simulink model "Greenhouse_Active_Passive_Solar_final"  (R2020b)
settings: Solver=VariableStepAuto  StartTime=0.0  StopTime=8759  RelTol=1e-3
libraries: simulink x1
settings Model: Creator=jkarenzi  LastModifiedBy=michelechamberlin

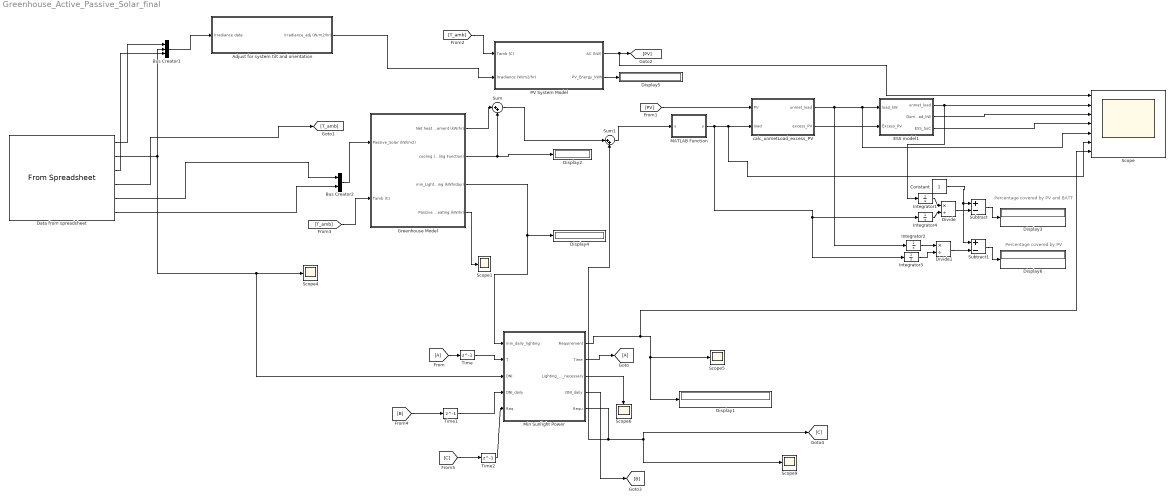
== system Greenhouse_Active_Passive_Solar_final ==
  note: Percentage covered by PV
  note: Percentage covered by PV and BATT
  Adjust for system tilt and orientation : Subsystem  TreatAsAtomicUnit=on  mask{P1=65, P2=65, P3=180}
      mask prompts: P1 "Latitude (degrees)"; P2 "System tilt (degrees)"; P3 "System Orientation (degrees)"
      mask init:
      | L = P1;
      | B = P2;
      | Z = P3;
  Bus Creator1 : BusCreator  Inputs=3
  Bus Creator2 : BusCreator  Inputs=2
  Constant : Constant
  Data from spreadsheet : FromSpreadsheet  FileName=C:\Users\michelechamberlin\Desktop\MicroFEWs\MATLAB Simulink\Tanana\GreenhouseData.xlsx  SheetName=GreenhouseData  Range=A1:G8761  SampleTime=1
  Display{1..6} (6 alike) : Display
  Divide : Product  Inputs=*/
  Divide1 : Product  Inputs=*/
  ESS model1 : Subsystem  TreatAsAtomicUnit=on  mask{P1=100, P2=100, P3=30, P4=90, P5=80}
      mask prompts: P1 "ESS Capacity"; P2 "Initial_SoC (%)"; P3 "Min_SoC (%)"; P4 "Max_SoC (%)"; P5 "Battery Efficieny (%)"
      mask init:
      | Bat_capacity = P1;
      | Init_SoC = P2;
      | min_SoC = P3;
      | max_SoC = P4;
      | bat_eff = P5;
  Greenhouse Model : Subsystem  mask{P1=60, P2=16, P3=750}
      mask prompts: P1 "Minimum inside temperature (F)"; P2 "Daily Artificial Lighting Hours"; P3 "Min. lighting requirements (fc)"
      mask init:
      | %Initialization
      | Tin = P1;
      | AL_hrs = P2;
      | min_lighting = P3;
  Integrator{1..4} (4 alike) : Integrator
  MATLAB Function : MATLAB Function  TreatAsAtomicUnit=on
  Min Sunlight Power : MATLAB Function  TreatAsAtomicUnit=on
  PV System Model : Subsystem  mask{DC=10, TC=-0.0037, MM=15, Inv=96}
      mask prompts: DC "DC system size (kW)"; TC "Temp coeff (%)"; MM "System losses (%)"; Inv "Inverter efficiency (%)"
      mask init:
      | %initiliaze the parameters
      | %PV System size
      | DC_kW = DC; %DC system size
      | T_coeff = TC; %temp coefficient
      | 
      | %define losses
      | L_modules = MM; %losses due to module mismatch
      | %L_dirt = LD; %Losses due to dirt
      | 
      | inv_eff = Inv; %inverter efficiency
  Scope : Scope  NumInputPorts=7
  Scope{1,4..6,9} (5 alike) : Scope
  Subtract : Sum  Inputs=+-
  Subtract1 : Sum  Inputs=+-
  Sum : Sum  Inputs=|++
  Sum1 : Sum  Inputs=|++
  Time : Delay  DelayLength=1  InitialCondition=0  SampleTime=1
  Time1 : Delay  DelayLength=1  InitialCondition=0  SampleTime=1
  Time2 : Delay  DelayLength=1  InitialCondition=0  SampleTime=1
  calc_unmetLoad_excess_PV : MATLAB Function  TreatAsAtomicUnit=on
  wires:
  Greenhouse Model/2(cooling (m3/s/m2) NEW: kW (Check cooling Function)) -> Sum/2, Display2/1
  Greenhouse Model/3(min_Lighting (kWh/day)) -> Min Sunlight Power/1(min_daily_lighting), Display4/1
  Bus Creator1/1 -> Adjust for system tilt and orientation/1(Irradiance data)
  Adjust for system tilt and orientation/1(Irradiance_adj (W/m2/hr)) -> PV System Model/2(Irradiance (W/m2/hr))
  PV System Model/2(PV_Energy_kWh) -> Display5/1
  PV System Model/1(AC (kW)) -> Scope/1, [PV]
  Data from spreadsheet/6 -> Bus Creator2/2
  Data from spreadsheet/5 -> Bus Creator2/1
  Data from spreadsheet/1 -> Bus Creator1/1
  Data from spreadsheet/2 -> Min Sunlight Power/3(DNI), Scope4/1, Bus Creator1/2
  Data from spreadsheet/3 -> Bus Creator1/3
  Data from spreadsheet/4 -> [T_amb]
  [T_amb] -> PV System Model/1(Tamb (C))
  Bus Creator2/1 -> Greenhouse Model/1(Passive_Solar (kW/m2))
  [T_amb] -> Greenhouse Model/2(Tamb (C))
  Greenhouse Model/4(Passive heating (kW/hr)) -> Scope1/1
  ESS model1/1(unmet_load) -> Integrator1/1, Scope/2
  [PV] -> calc_unmetLoad_excess_PV/1(PV)
  calc_unmetLoad_excess_PV/2(excess_PV) -> ESS model1/2(Excess_PV)
  Greenhouse Model/1(Net heat requirement (kW/hr)) -> Sum/1
  ESS model1/2(Dump_load_kW) -> Scope/3
  ESS model1/3(ESS_SoC) -> Scope/4
  Min Sunlight Power/1(Requirement) -> Display1/1, Scope5/1, Scope/7
  Min Sunlight Power/3(Lighting_Wh_necessary) -> Scope6/1
  [A] -> Time/1
  Time/1 -> Min Sunlight Power/2(T)
  Min Sunlight Power/2(Time) -> [A]
  Sum1/1 -> MATLAB Function/1(u)
  Sum/1 -> Sum1/1
  MATLAB Function/1(y) -> Integrator3/1, Integrator4/1, Scope/6, calc_unmetLoad_excess_PV/2(load)
  Integrator1/1 -> Divide/1
  Integrator4/1 -> Divide/2
  Divide/1 -> Subtract/2
  Integrator2/1 -> Divide1/1
  Divide1/1 -> Subtract1/2
  Integrator3/1 -> Divide1/2
  calc_unmetLoad_excess_PV/1(unmet_load) -> Integrator2/1, Scope/5, ESS model1/1(load_kW)
  Constant/1 -> Subtract/1, Subtract1/1
  Subtract/1 -> Display3/1
  Subtract1/1 -> Display6/1
  Min Sunlight Power/4(DNI_daily) -> [B]
  [B] -> Time1/1
  Time1/1 -> Min Sunlight Power/4("DNI_daily ")
  Time2/1 -> Min Sunlight Power/5(Req)
  [C] -> Time2/1
  Min Sunlight Power/5(Requ) -> Scope9/1, [C], Sum1/2

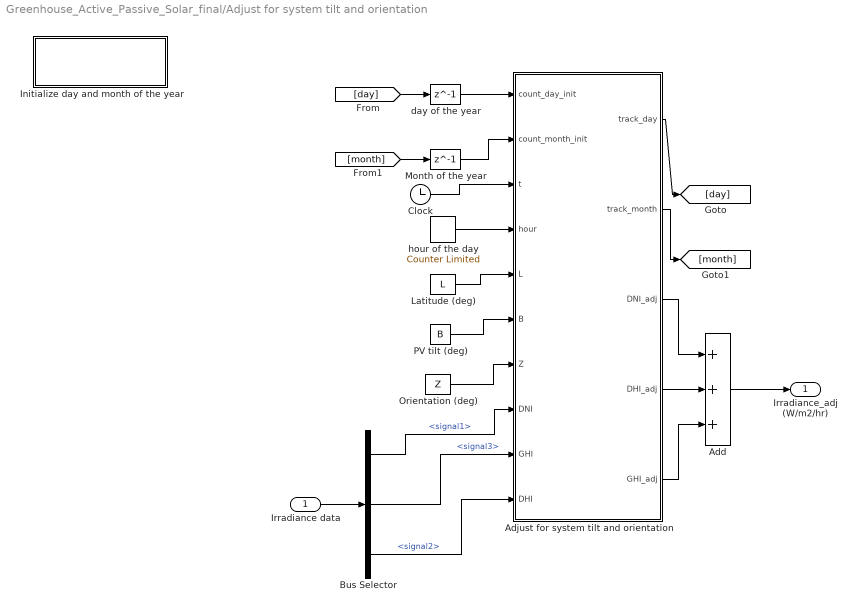
== system Greenhouse_Active_Passive_Solar_final/Adjust for system tilt and orientation ==
  Irradiance data : Inport
  Add : Sum  Inputs=+++
  Adjust for system tilt and orientation : MATLAB Function  TreatAsAtomicUnit=on
  Bus Selector : BusSelector  OutputSignals=signal1,signal3,signal2
  Clock : Clock
  Initialize day and month of the year : Subsystem  TreatAsAtomicUnit=on
  Latitude (deg) : Constant  Value=L
  Month of the year : Delay  DelayLength=1  InitialCondition=0  SampleTime=1
  Orientation (deg) : Constant  Value=Z
  PV tilt (deg) : Constant  Value=B
  day of the year : Delay  DelayLength=1  InitialCondition=0  SampleTime=1
  hour of the day : simulink/Sources/Counter Limited  uplimit=24  tsamp=1
  Irradiance_adj (W/m2/hr) : Outport
  wires:
  [month] -> Month of the year/1
  Adjust for system tilt and orientation/1(track_day) -> [day]
  Adjust for system tilt and orientation/5(GHI_adj) -> Add/3
  day of the year/1 -> Adjust for system tilt and orientation/1(count_day_init)
  PV tilt (deg)/1 -> Adjust for system tilt and orientation/6(B)
  Month of the year/1 -> Adjust for system tilt and orientation/2(count_month_init)
  Adjust for system tilt and orientation/2(track_month) -> [month]
  hour of the day/1 -> Adjust for system tilt and orientation/4(hour)
  Clock/1 -> Adjust for system tilt and orientation/3(t)
  [day] -> day of the year/1
  Orientation (deg)/1 -> Adjust for system tilt and orientation/7(Z)
  Adjust for system tilt and orientation/3(DNI_adj) -> Add/1
  Adjust for system tilt and orientation/4(DHI_adj) -> Add/2
  Latitude (deg)/1 -> Adjust for system tilt and orientation/5(L)
  Add/1 -> Irradiance_adj (W/m2/hr)/1
  Irradiance data/1 -> Bus Selector/1
  Bus Selector/1 -> Adjust for system tilt and orientation/8(DNI)  "<signal1>"
  Bus Selector/2 -> Adjust for system tilt and orientation/9(GHI)  "<signal3>"
  Bus Selector/3 -> Adjust for system tilt and orientation/10(DHI)  "<signal2>"

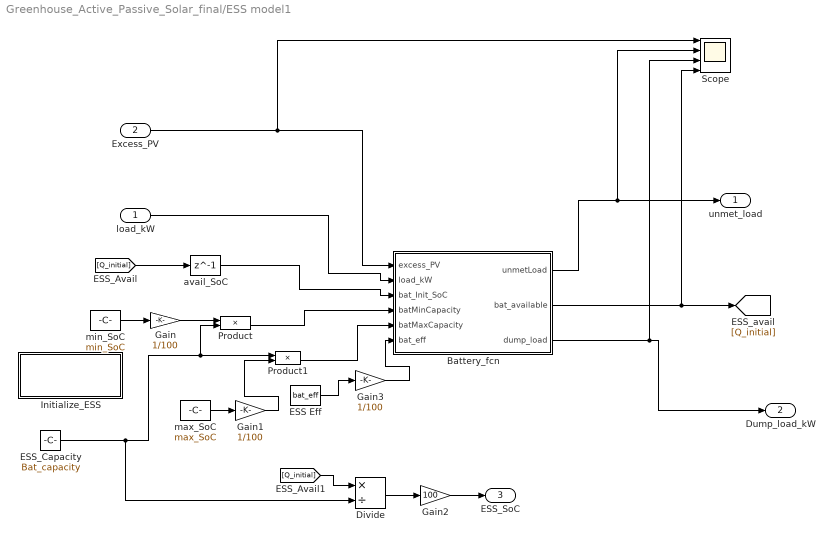
== system Greenhouse_Active_Passive_Solar_final/ESS model1 ==
  load_kW : Inport
  Excess_PV : Inport  Port=2
  Battery_fcn : MATLAB Function  TreatAsAtomicUnit=on
  Divide : Product  Inputs=*/
  ESS Eff : Constant  Value=bat_eff
  "ESS_Capacity " : Constant  Value=Bat_capacity
  Gain : Gain  Gain=1/100
  Gain1 : Gain  Gain=1/100
  Gain2 : Gain  Gain=100
  Gain3 : Gain  Gain=1/100
  Initialize_ESS : Subsystem  TreatAsAtomicUnit=on
  Product : Product
  Product1 : Product
  Scope : Scope  NumInputPorts=4
  avail_SoC : Delay  DelayLength=1  InitialCondition=0  SampleTime=1
  max_SoC : Constant  Value=max_SoC
  min_SoC : Constant  Value=min_SoC
  unmet_load : Outport
  Dump_load_kW : Outport  Port=2
  ESS_SoC : Outport  Port=3
  wires:
  Excess_PV/1 -> Scope/1, Battery_fcn/1(excess_PV)
  avail_SoC/1 -> Battery_fcn/3(bat_Init_SoC)
  Battery_fcn/1(unmetLoad) -> Scope/2, unmet_load/1
  [Q_initial] -> avail_SoC/1
  max_SoC/1 -> Gain1/1
  min_SoC/1 -> Gain/1
  Gain/1 -> Product/1
  Product/1 -> Battery_fcn/4(batMinCapacity)
  Product1/1 -> Battery_fcn/5(batMaxCapacity)
  Gain1/1 -> Product1/2
  load_kW/1 -> Battery_fcn/2(load_kW)
  Battery_fcn/2(bat_available) -> Scope/4, [Q_initial]
  Battery_fcn/3(dump_load) -> Scope/3, Dump_load_kW/1
  ESS Eff/1 -> Gain3/1
  Gain3/1 -> Battery_fcn/6(bat_eff)
  "ESS_Capacity "/1 -> Divide/2, Product1/1, Product/2
  [Q_initial] -> Divide/1
  Divide/1 -> Gain2/1
  Gain2/1 -> ESS_SoC/1

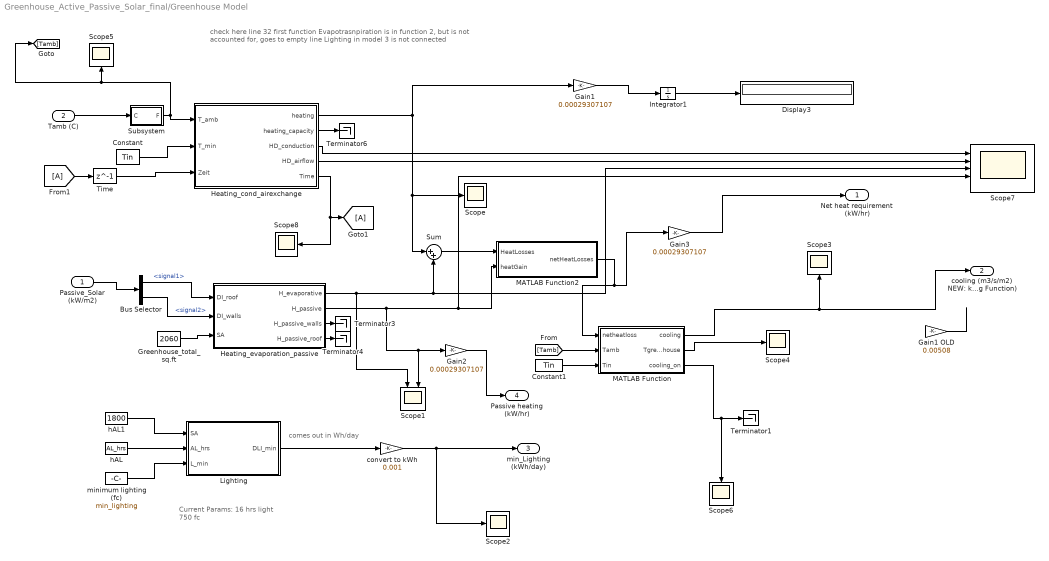
== system Greenhouse_Active_Passive_Solar_final/Greenhouse Model ==
  note: Current Params:
      | 16 hrs light
      | 750 fc
  note: comes out in Wh/day
  note: check here line 32 first function
      | Evapotrasnpiration is in function 2, but is not accounted for, goes to empty line
      | Lighting in model 3 is not connected
  Passive_Solar (kW/m2) : Inport
  Tamb (C) : Inport  Port=2
  Bus Selector : BusSelector  OutputSignals=signal1,signal2
  Constant : Constant  Value=Tin
  Constant1 : Constant  Value=Tin
  Display3 : Display
  Gain1 : Gain  Gain=0.00029307107
  Gain1 OLD : Gain  Gain=0.00508
  Gain2 : Gain  Gain=0.00029307107
  Gain3 : Gain  Gain=0.00029307107
  Greenhouse_total_sq.ft : Constant  Value=2060
  Heating_cond_airexchange : MATLAB Function  TreatAsAtomicUnit=on
  Heating_evaporation_passive : MATLAB Function  TreatAsAtomicUnit=on
  Integrator1 : Integrator
  Lighting : MATLAB Function  TreatAsAtomicUnit=on
  MATLAB Function : MATLAB Function  TreatAsAtomicUnit=on
  MATLAB Function2 : MATLAB Function  TreatAsAtomicUnit=on
  Scope{,2..6,8} (7 alike) : Scope
  Scope1 : Scope  NumInputPorts=2
  Scope7 : Scope  NumInputPorts=5
  Subsystem : Subsystem
  Sum : Sum  Inputs=|++
  Terminator{1,3..4,6} (4 alike) : Terminator
  Time : Delay  DelayLength=1  InitialCondition=0  SampleTime=1
  convert to kWh : Gain  Gain=0.001
  hAL : Constant  Value=AL_hrs
  hAL1 : Constant  Value=1800
  minimum lighting (fc) : Constant  Value=min_lighting
  Net heat requirement (kW/hr) : Outport
  cooling (m3/s/m2) NEW: kW (Check cooling Function) : Outport  Port=2
  min_Lighting (kWh/day) : Outport  Port=3
  Passive heating (kW/hr) : Outport  Port=4
  wires:
  Heating_evaporation_passive/4(H_passive_roof) -> Terminator4/1
  Heating_evaporation_passive/3(H_passive_walls) -> Terminator3/1
  Bus Selector/2 -> Heating_evaporation_passive/2(DI_walls)  "<signal2>"
  Bus Selector/1 -> Heating_evaporation_passive/1(DI_roof)  "<signal1>"
  Passive_Solar (kW/m2)/1 -> Bus Selector/1
  convert to kWh/1 -> Scope2/1, min_Lighting (kWh/day)/1
  Lighting/1(DLI_min) -> convert to kWh/1
  hAL1/1 -> Lighting/1(SA)
  minimum lighting (fc)/1 -> Lighting/3(L_min)
  MATLAB Function/3(cooling_on) -> Terminator1/1, Scope6/1
  MATLAB Function/2(Tgreenhouse) -> Scope4/1
  Heating_cond_airexchange/2(heating_capacity) -> Terminator6/1
  Constant1/1 -> MATLAB Function/3(Tin)
  [Tamb] -> MATLAB Function/2(Tamb)
  Heating_evaporation_passive/1(H_evaporative) -> Scope1/1, Sum/2, Scope7/3
  hAL/1 -> Lighting/2(AL_hrs)
  Subsystem/1(F) -> [Tamb], Scope5/1, Heating_cond_airexchange/1(T_amb)
  Tamb (C)/1 -> Subsystem/1(C)
  MATLAB Function2/1(netHeatLosses) -> MATLAB Function/1(netheatloss), Gain3/1
  Heating_evaporation_passive/2(H_passive) -> Gain2/1, Scope1/2, Scope7/4, MATLAB Function2/2(heatGain)
  Heating_cond_airexchange/1(heating) -> Gain1/1, Sum/1, Scope/1
  Greenhouse_total_sq.ft/1 -> Heating_evaporation_passive/3(SA)
  Constant/1 -> Heating_cond_airexchange/2(T_min)
  Gain3/1 -> Net heat requirement (kW/hr)/1
  MATLAB Function/1(cooling) -> cooling (m3/s/m2) NEW: kW (Check cooling Function)/1, Scope3/1
  Gain1 OLD/1 -> ?
  Gain2/1 -> Passive heating (kW/hr)/1
  Sum/1 -> MATLAB Function2/1(HeatLosses)
  Heating_cond_airexchange/3(HD_conduction) -> Scope7/1
  Heating_cond_airexchange/4(HD_airflow) -> Scope7/2
  Time/1 -> Heating_cond_airexchange/3(Zeit)
  [A] -> Time/1
  Heating_cond_airexchange/5(Time) -> Scope8/1, [A]
  Gain1/1 -> Integrator1/1
  Integrator1/1 -> Display3/1

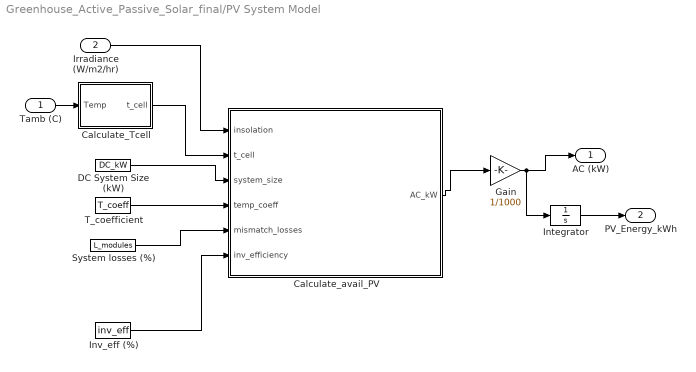
== system Greenhouse_Active_Passive_Solar_final/PV System Model ==
  Tamb (C) : Inport
  Irradiance (W/m2/hr) : Inport  Port=2
  Calculate_Tcell : MATLAB Function  TreatAsAtomicUnit=on
  Calculate_avail_PV : MATLAB Function  TreatAsAtomicUnit=on
  DC System Size (kW) : Constant  Value=DC_kW
  Gain : Gain  Gain=1/1000
  Integrator : Integrator
  Inv_eff (%) : Constant  Value=inv_eff
  System losses (%) : Constant  Value=L_modules
  T_coefficient : Constant  Value=T_coeff
  AC (kW) : Outport  VectorParamsAs1DForOutWhenUnconnected=off
  PV_Energy_kWh : Outport  Port=2  VectorParamsAs1DForOutWhenUnconnected=off
  wires:
  Gain/1 -> AC (kW)/1, Integrator/1
  Integrator/1 -> PV_Energy_kWh/1
  Calculate_avail_PV/1(AC_kW) -> Gain/1
  Irradiance (W/m2/hr)/1 -> Calculate_avail_PV/1(insolation)
  Calculate_Tcell/1(t_cell) -> Calculate_avail_PV/2(t_cell)
  Tamb (C)/1 -> Calculate_Tcell/1(Temp)
  DC System Size (kW)/1 -> Calculate_avail_PV/3(system_size)
  T_coefficient/1 -> Calculate_avail_PV/4(temp_coeff)
  System losses (%)/1 -> Calculate_avail_PV/5(mismatch_losses)
  Inv_eff (%)/1 -> Calculate_avail_PV/6(inv_efficiency)

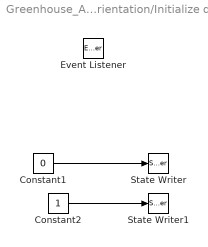
== system Greenhouse_Active_Passive_Solar_final/Adjust for system tilt and orientation/Initialize day and month of the year ==
  Constant1 : Constant  Value=0
  Constant2 : Constant
  Event Listener : EventListener  DisableCoverage=on  EventName=reset
  State Writer : StateWriter  StateOwnerBlock=../../day of the year
  State Writer1 : StateWriter  StateOwnerBlock=../../Month of the year
  wires:
  Constant2/1 -> State Writer1/1
  Constant1/1 -> State Writer/1

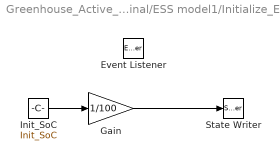
== system Greenhouse_Active_Passive_Solar_final/ESS model1/Initialize_ESS ==
  Event Listener : EventListener  DisableCoverage=on  EventName=reset
  Gain : Gain  Gain=1/100
  Init_SoC : Constant  Value=Init_SoC
  State Writer : StateWriter  StateOwnerBlock=../../avail_SoC
  wires:
  Init_SoC/1 -> Gain/1
  Gain/1 -> State Writer/1

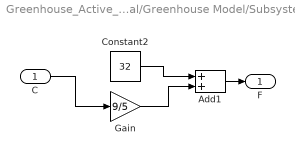
== system Greenhouse_Active_Passive_Solar_final/Greenhouse Model/Subsystem ==
  C : Inport
  Add1 : Sum
  Constant2 : Constant  Value=32
  Gain : Gain  Gain=9/5
  F : Outport
  wires:
  Add1/1 -> F/1
  C/1 -> Gain/1
  Gain/1 -> Add1/2
  Constant2/1 -> Add1/1

== matlab function Greenhouse_Active_Passive_Solar_final/Greenhouse Model/Heating_cond_airexchange ==
  data: T_amb input; heating output; T_min input; heating_capacity output; HD_conduction output; HD_airflow output; Zeit input; Time output
function [heating,heating_capacity,HD_conduction,HD_airflow,Time]   = fcn(T_amb,T_min,Zeit)
%function estimates the heating requirements of the greenhouse
S_ceil = 430; %south facing ceiling (assume at an angle of 45deg)in sq.ft
N_ceil = 430; %north facing ceiling in sq.ft
E_W_S = 1200; %total square footage of the S,E,W walls
N = 960; %totall square footage of the N wall
floor = 1800; %floor area
%U values
%make night insolation (different U values at night, due to night insulation from 2000 to 0600)
if rem(Zeit,24)<8 || rem(Zeit,24)>20 %nighttime, reduction of 0.2 BTU/hr/ft/other freedom units
    U_north = 0.2; %suggested by Dan Sambor
    U_south = 0.3; %for all other walls: 0.5 double pane glass, 0.33 triple pane (subtract 0.2 for night insulation)
    U_floor = 0.1; %concrete floor
else %daytime
    U_north = 0.2;
    U_south = 0.5; %for all other walls
    U_floor = 0.1; %concrete floor
end
    
%air exchange
C = 1.5; %Air exchange per hour depends on the construction material. value ranges from 0.5-1.5
H = 10; %Assume a height of 10ft
V = floor*H; %volume of the greenhouse
heating_capacity = (U_south * E_W_S + U_north*N + (S_ceil + N_ceil) * U_south + floor * U_floor + 0.02 * C *V)*T_min; %% Conduction and air excange

if(T_amb>T_min) % check if ambient temp is not greater than min_set temperature
    heating=0;
    heating_conduction = 0;
    heating_evapotranspiration = 0;
    
else

%heat losses (perimeter)
heating_S_E_W = U_south * E_W_S* abs(T_amb-T_min);
heating_n = U_north*N*abs(T_amb-T_min);
heating_ceil = (S_ceil + N_ceil) * U_south * abs(T_amb-T_min);
heating_floor = floor * U_floor *abs(T_amb-T_min);
heating_conduction = heating_S_E_W + heating_n + heating_ceil + heating_floor;

heating_evapotranspiration = 0.02 * C *V*abs(T_amb-T_min); %% HERE isn't this air exchange loss????

heating = heating_conduction + heating_evapotranspiration;
end

HD_airflow = heating_evapotranspiration
HD_conduction = heating_conduction
Time = Zeit+1

== matlab function Greenhouse_Active_Passive_Solar_final/Greenhouse Model/Heating_evaporation_passive ==
  data: DI_roof input; DI_walls input; H_evaporative output; SA input; H_passive output; H_passive_walls output; H_passive_roof output
function [H_evaporative,H_passive,H_passive_walls,H_passive_roof] = fcn(DI_roof,DI_walls,SA)
%function estimates heat losses due to evaporation
%Passive Solar Heating
%T: Transmittance value

%SA: Surface Area
%DLI: Solar Radiation intensity on a horizontal surface (1kWh/m2 = 316.998
%BTU/ft2)
%FC: Floor use factor - ratio of ground covered by plants to total ground area


S_ceil = (430)*0.0929; %south facing ceiling (assume at an angle of 45deg)in sq.m
N_ceil = S_ceil; %north facing ceiling in sq.ft
E_W_S = (1200)*0.0929; %total square footage of the S,E,W walls
N = (960)*0.0929; %totall square footage of the N wall
T = 0.7; %Assume a transmittance value of 0.7
FF = 0.9; %Assuming a floor use factor
%total solar gain does not account for the north facing wall since it is
%opaque
H_passive_walls = DI_walls * (E_W_S)*0.3156*T;
H_passive_roof = (DI_roof*S_ceil*2)*0.3156*T;
H_passive = H_passive_walls + H_passive_roof;
H_evaporative = 0.3 * FF * H_passive;


% DLI = (((E_W_S/2)*S)+(S_ceil*S_45)+((E_W_S/4)*E) + ((E_W_S/4)*W) + (N_ceil*N_45));
% DLI = DLI*0.3156*T;
%DLI = TotalSolarGain*0.3156; %converting to BTU/hr
% H_passive = DLI;

== matlab function Greenhouse_Active_Passive_Solar_final/Greenhouse Model/Lighting ==
  data: SA input; AL_hrs input; L_min input; DLI_min output
function DLI_min = fcn(SA,AL_hrs,L_min)

%SA: Surface area of the greenhouse
%L_min: minimal lighting requirements
%AL_hrs: hours of artificial lighting required (depends on the crop)
%DLI_natural: Amount of natural sunlight available
%estimate min. artificial lighting required
SA = SA*0.0929; %convert to sq.m
DLI_min = AL_hrs*SA*(L_min*0.01609); %% fc to W/m^2 conversion is 0.01609
%Lmin is fc

== matlab function Greenhouse_Active_Passive_Solar_final/Greenhouse Model/MATLAB Function ==
  data: netheatloss input; Tamb input; cooling output; Tgreenhouse output; cooling_on output; Tin input
function [cooling,Tgreenhouse,cooling_on] = fcn(netheatloss,Tamb,Tin)
%cooling requirements of the greenhouse

S_ceil = 430; %south facing ceiling (assume at an angle of 45deg)in sq.ft
N_ceil = 430; %north facing ceiling in sq.ft
E_W_S = 1200; %total square footage of the S,E,W walls
N = 960; %totall square footage of the N wall
floor = 1800; %floor area
%U values
U_north = 0.8; 
U_south = 0.5; %for all other walls
U_floor = 0.1; %concrete floor
H = 10; %Assume a height of 10ft
V = floor*H; %volume of the greenhouse
C = 1.5; %Air exchange per hour depends on the construction material. value ranges from 0.5-1.5
% if(netheatloss<0)
%     delT = 0;
% else
   delT = abs(netheatloss/( U_south*E_W_S  + U_north*N + (S_ceil + N_ceil)*U_south + floor*U_floor + 0.02*C*V));
%end
cooling = floor * 8; %assume 8cfm/ft2 (m^3/ft^2) MJC: this is the cooling demand in CFM.
% Internet search for greenhouse fans shows a 1HP motor fan provides
% approx. 20'000 cfm. In this specific case, with cooling=14400 cfm
% required, this fan generously satisfies the cooling requiremnt and for
% power -> 1mech HP = 0.745 kW, but accounting for efficiency, it is more
% like 1.008kW
%https://www.thepoultrysite.com/articles/motor-size-is-poor-indicator-of-fan-power-usage#:~:text=Just%20taking%20into%20account%20motor,power%20into%20the%20fan%20motor.&text=A%20third%20factor%20is%20the%20a%20motor's%20service%20factor.




Tgreenhouse = delT+(Tamb);
if((Tin - Tgreenhouse)<-5) %MJC: Cooling is on if Tgreen > (Tin+7). Changed value to 5 (Ideally, GH has 80-85F
    cooling_on = 1;
else
    cooling_on = 0;
end

%RENEW Cooling Variable to be the Cooling demand in kW
cooling = cooling_on*1.008

== matlab function Greenhouse_Active_Passive_Solar_final/Greenhouse Model/MATLAB Function2 ==
  data: HeatLosses input; heatGain input; netHeatLosses output
function netHeatLosses   = fcn(HeatLosses,heatGain)
%function checks the heat required (demand) for the greenhouse

netHeatLosses = HeatLosses - heatGain;
% if(netHeatLosses<0 )
%     netHeatLosses = 0;
%     
% end

== matlab function Greenhouse_Active_Passive_Solar_final/MATLAB Function ==
  data: u input; y output
function y = fcn(u)


if u<0
    u=0
end

y = u;

== matlab function Greenhouse_Active_Passive_Solar_final/Min Sunlight Power ==
  data: min_daily_lighting input; T input; DNI input; Requirement output; Time output; Lighting_Wh_necessary output; DNI_daily input; DNI_daily output; Req input; Requ output
function [Requirement,Time, Lighting_Wh_necessary,DNI_daily,Requ]    = fcn(min_daily_lighting, T, DNI,DNI_daily, Req)


%min_daily_lighting is min daily light in kWh/day (alreadt adapted to area)
%DNI is Direct Normal irradiance in W/m^2
%Requ, Req, Time, and T are all variables that get passed to next time
%This is to 'store information'. Requ and Req are passed, in order to
%compare the daily requirement with the sum of the daily solar irradiance
%(this requires the total sum of the hourly solar data to be passed on)

SA = 1800
SA = SA*0.0929; %convert to sq.m
Sunlight_tot = DNI*SA % from W/m^2 to W
%0.41 is the sunlight to PAR and 0.8 is the transmissivity of the greenhouse
Lighting_Wh_necessary= min_daily_lighting/24*1000% from kWh per day average Wattage (Wh per hour)
%Now overwrite the input value, because it is in foot-candles in the matlab function and that just
%makes things more complicated, so we want our number in Wh/m2 as done
%below (for high-light requirement plants
Lighting_Wh_necessary=3313 %Wh/m2/day % computed on separate spreadsheet, resulting from plant requirement of 18 mol/m2/day
Lighting_Wh_necessary= 3313*SA % Wh/day % daily necessary solar radiation energy (converteed with 0.8 transmissivity and 0.41 is the sunlight to PAR 

Requirement=0

%if (T<2880 || T>6450) %given assumption over the daily spread, only do this during non summer months
counter=1
if T==0
    DNI_daily=0
    Requirement=0
end

% This is a little weird, but if one simulates timeseries in Simulink,
% that's what you get!

if rem(T,24) ==23 % At the 'end' of the day count to see how much cumulative DNI deviates from required DNI (required DNI is already corrected for PAR/Sunlight and transmissivity,, etc.....)
    % Requirement is here 'allocated' to final hour of the day, due to the
    % simulation being done in Simulink. In terms of total DNI required, that is
    % fine, but for PV coverage, the problem is solved by dividing the
    % required/missing DNI of day X  by 24 (hours) and placing it as an 
    %electrical load (by means of mol/W(el) of LED) to each hour of day X+1 (I know...), i
    counter=0 %reset counter
     if (DNI_daily*SA) <Lighting_Wh_necessary
        Requirement = Lighting_Wh_necessary - (DNI_daily*SA)%missing Wh of solar radiation
        Requirement = Requirement/184.1 %factor to get from Wh solar to mol PAR  % this value is in mol/day per entire greenhouse
        Requirement= Requirement/2.3508*384 % 2.3508 mol/hour from a red-blue LED that uses 384 W electric % this unit is in Wh/day (it cumulates the entire daily demand into one hour, but for the energy demand, this is not a problem. It is better than averaging the daily plant demand and finding the corresponding hourly lighting requirement
     else
        Requirement=0
       
    end
    
    DNI_daily=0
    
    
end

if rem(T,24)==0
    counter=1 %restart counter
    DNI_daily=0
    Requirement=0 %reset
    Requ = 0 %reset at the end of the day
   

end

if counter == 1
    DNI_daily=DNI_daily+DNI % get cumulative sum of DNI to compare it to the DLI requirement of lamps
    
    Requirement=0
  
end



        
    
%else
    %Requirement=0
%end

Requirement= Requirement/1000 % to kWh/h
if Requirement>0
    Requ=Requirement/24 %Due to the step-by-step nature of Simulink,there is no instantaneous distribution of the artificial lighting demand, because that has to be determined first
    %So, 
else
    Requ=Req
end
    
    
Time = T+1

== matlab function Greenhouse_Active_Passive_Solar_final/calc_unmetLoad_excess_PV ==
  data: PV input; load input; unmet_load output; excess_PV output
function [unmet_load,excess_PV] = fcn(PV,load)
%Calculate how PV is available and supply the load
if (PV>load)
    unmet_load = 0;
    excess_PV = PV-load;
elseif (PV==load)
    unmet_load = 0;
    excess_PV = 0;
else 
    unmet_load = load-PV;
    excess_PV = 0;
end

== matlab function Greenhouse_Active_Passive_Solar_final/ESS model1/Battery_fcn ==
  data: excess_PV input; unmetLoad output; load_kW input; bat_Init_SoC input; batMinCapacity input; batMaxCapacity input; bat_eff input; bat_available output; dump_load output
function [ unmetLoad,bat_available,dump_load] = batt_fcn(excess_PV,load_kW,bat_Init_SoC,batMinCapacity,batMaxCapacity,bat_eff)
%if generation meets demand, no unmentload, energy storage unchanged, no
%excess renewable
%Here load_kW represents unmet load
bat_available = bat_Init_SoC;
%if load is greater than generation, use battery to cover the unmet load
if(load_kW > 0)
    %Check how much energy the battery has. If at minimum, send unmet
    %load to diesel
    if(bat_available<=batMinCapacity)
        bat_available = batMinCapacity;
        unmetLoad = load_kW;
        dump_load = 0 ;
        
        %If there's power in the battery, meet the load till the minimum is reached. then send
        %rest to the diesel
    elseif ((bat_available>batMinCapacity)&& (load_kW>(bat_available-batMinCapacity))) %batt avail greater bat min cap
        %  if(load_kW>(bat_available-batMinCapacity)) %unmet load > avail battery
        bat_available = batMinCapacity;
        unmetLoad = load_kW - (bat_Init_SoC - batMinCapacity); %%here should be load_kW-(bat_available-batMinCapacity)????
        dump_load = 0 ;
        
        %neglect self discharge rate
    else
        bat_available = bat_Init_SoC - load_kW;
        unmetLoad = 0;
        dump_load = 0 ;
    end
    % end
    %if generation meets demand and there's no excess PV
elseif ((load_kW == 0)&& (excess_PV ==0))
    bat_available =  bat_Init_SoC;
    unmetLoad = 0;
    dump_load = 0 ;
    %if there is excess PV, charge the ESS. Ignoring the self discharge rates
elseif(excess_PV >0)
    
    
    %  PVExcess = P_charge_kW - load_kW;
    if((bat_available+excess_PV/bat_eff)>=batMaxCapacity)
        dump_load = excess_PV-((batMaxCapacity-bat_available)/(bat_eff));%%MJC line was: dump_load = excess_PV
        bat_available = batMaxCapacity;
        unmetLoad = 0;
    else
        bat_available =  bat_available + excess_PV *(bat_eff);
        unmetLoad = 0;
        dump_load = 0;
    end
    
else
    bat_available = bat_Init_SoC;
    unmetLoad = 0;
    dump_load = 0;
end
end

== matlab function Greenhouse_Active_Passive_Solar_final/Adjust for system tilt and orientation/Adjust for system tilt and orientation ==
  data: track_day output; track_month output; count_day_init input; count_month_init input; t input; hour input; L input; B input; Z input; DNI input; DNI_adj output; DHI_adj output; GHI input; DHI input; GHI_adj output
function [track_day, track_month, DNI_adj,DHI_adj,GHI_adj] = fcn(count_day_init,count_month_init,t,hour,L,B,Z,DNI,GHI,DHI)

%L: Latitude
%B: tilt
%Z: surface azimuth
hour = double(hour);

m=[0 31 59 90 120 151 181 212 243 273 304 334]; %days in the year

if (mod(t,24) ==0)
track_day = count_day_init + 1;
else
  track_day = count_day_init; 
end

if(mod(t,730) == 0)
 track_month = count_month_init + 1;
else
    track_month = count_month_init;
end

n= m(track_month)+ track_day;

%declination angle
declination_angle = 23.45*sin(360*(284+n)/365*pi/180); %see equ(1)   
d=declination_angle*pi/180; 

%hour angle
hour_angle = (hour-12)*15; %see equ(2)      
h=hour_angle*pi/180; 

%altitude angle
Altitude_angle = asin(sin(L)*sin(d)+cos(L)*cos(d)*cos(h))*180/pi; %see equ(3)
a=Altitude_angle*pi/180;

Solar_zenith_angle = 90-Altitude_angle;

phi =Solar_zenith_angle*pi/180; 
Solar_azimuth_angle= asin(cos(d)*sin(h)/cos(a))*180/pi; %see equ(4)
z =Solar_azimuth_angle*pi/180; 
 
L = L*180/pi;
Z = Z*180/pi;
B = B*180/pi;

Incidence_angle = acos(sin(L)*sin(d)*cos(B)- cos(L)*sin(d)*sin(B)*cos(Z)+ cos(L)*cos(d)*cos(h)*cos(B)...
+ sin(L)*cos(d)*cos(h)*sin(B)*cos(Z)+cos(d) *sin(h)*sin(B)*sin(Z))*180/pi; %see equ(5) 
theta =Incidence_angle*pi/180; 
%RB=cos(theta)/cos(phi); %see equ(6) 
HSRC = [ acos(complex((-tan(L)*tan(d)))) acos(complex((-tan(L-B)*tan(d))))];
HSRC = min(HSRC);
RB = (cos(L-B)*cos(d)*sin(HSRC) + HSRC*sin(L-B)*sin(d)) /(cos(L)*cos(d)*sin(HSRC) + HSRC*sin(L)*sin(d));
    
DNI_adj = abs(cos(theta))*DNI;
DHI_adj = (1+cos(B))/2*DHI;
GHI_adj = (1-cos(B))/2 * GHI;


end

== matlab function Greenhouse_Active_Passive_Solar_final/PV System Model/Calculate_Tcell ==
  data: Temp input; t_cell output
function t_cell  = T_cell(Temp)
%function reads the ambient temperature in deg. celcius and calculates the
%cell temperature
NOCT = 47; %Nominal Operating Cell Temperature
A_Temp = 20; %Ambient Temperature under NOCT
Solar_Irr = 0.8; %Solar Irrandiance of 0.8kW/m2
t_cell = Temp + ((NOCT-A_Temp)/Solar_Irr)*1; %Estimating Cell Temperature at 1-sun

== matlab function Greenhouse_Active_Passive_Solar_final/PV System Model/Calculate_avail_PV ==
  data: insolation input; AC_kW output; t_cell input; system_size input; temp_coeff input; mismatch_losses input; inv_efficiency input
function AC_kW = Solar_PV(insolation,t_cell,system_size, temp_coeff, mismatch_losses,inv_efficiency)

%function approximates the DC, AC, and energy (Kwh) solar PV Output using the
%peak sun hours approach as outlined in the Gilbert M. Masters 'Renewable and
%Efficient Electric Power Systems'.
%tcell: cell temperature
%system_size: DC kW system size
%insolation: kWh/m2/day or (hrs/day) of full sun available


if (insolation<0) %Check for insolation/Irradiance value is less than zero
    insolation = 0; 
end
DC_Power_kW = insolation*system_size *(1-temp_coeff*(t_cell-25));
%DC_Power_kW = system_size*(1-temp_coeff*(t_cell-25)); % Calculate DC Power using the new cell temperature
AC_kW = DC_Power_kW*(1-(mismatch_losses/100))*(inv_efficiency/100); %calculate AC Power accounting for losses


%kWh_output_AC = AC_kW *insolation; %hrs/day of full sun using the peak-sun hours
%PV_kWh = kWh_output_AC;
%PV_kWh = kWh_output_AC * 30; %monthly Output (Assume 30 days for 1 full month)
